simulink model "untitled3"  (R2023a)
settings: Solver=FixedStepAuto  StartTime=0.0  StopTime=3  FixedStep=1e-5  RelTol=1e-3
undefined symbols (not defined in the file): J, KT, La, Ra, UaN
libraries: spsMosfetLib x8, spsDCVoltageSourceLib x2, simulink x2, spsVoltageMeasurementLib x2, spsDCMachineLib x1, sps_lib x1
settings Model: Creator=luand  LastModifiedBy=luand

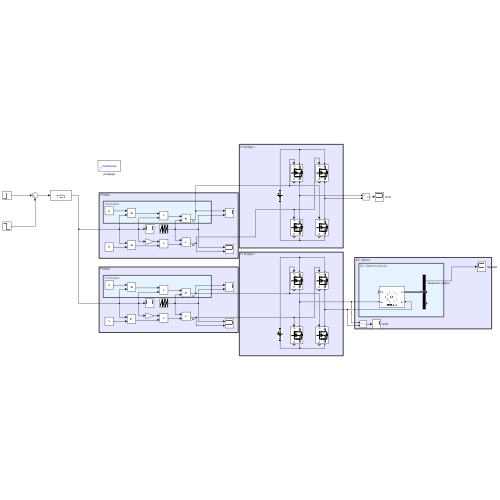
[thumbnail: Simulink's stored preview of the top-level diagram]
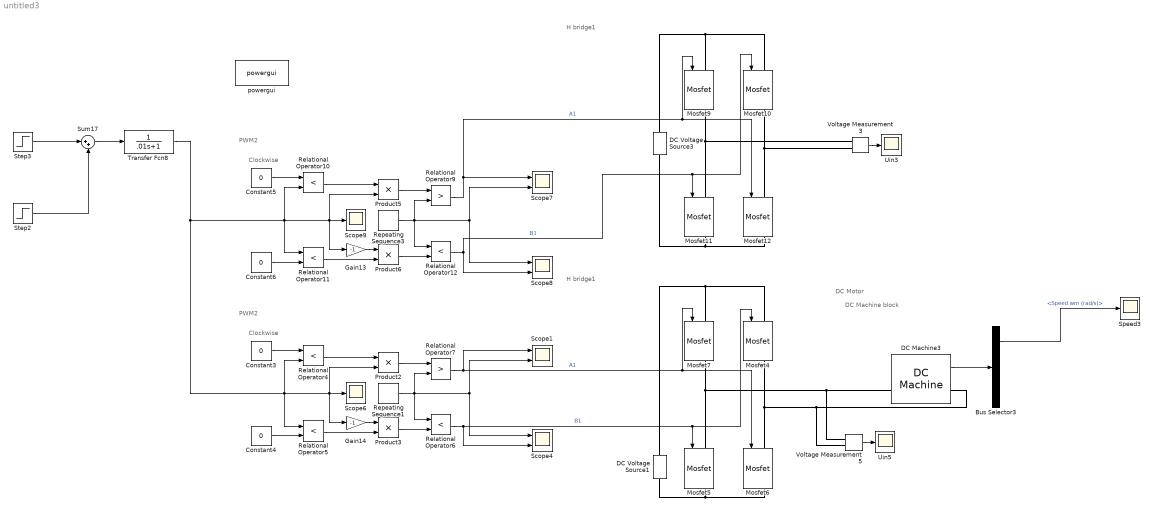
== system untitled3 ==
  note: PWM2
  note: Clockwise
  note: DC Machine block
  note: DC Motor
  note: PWM2
  note: H bridge1
  note: Clockwise
  note: H bridge1
  Bus Selector3 : BusSelector  OutputSignals=Speed wm (rad/s),Armature current ia (A),Electrical torque Te (n m)
  Constant{3..6} (4 alike) : Constant  Value=0
  DC Machine3 : spsDCMachineLib/DC Machine  PresetModel=No  MechanicalLoad=Torque TL  FieldType=Permanent magnet  ShowDetailedParameters=on  MeasurementBus=off  RLa=[ Ra La ]  RLf="[ 240  120]"  Laf=1.8  MachineConstant=Torque constant (N.m/A)  Ke=1.8  Kt=KT  J=J  Bm=0  Tf=0  w0=0  Ifinit=1  TsPowergui=0  TsBlock=-1
  DC Voltage Source1 : spsDCVoltageSourceLib/DC Voltage Source  Amplitude=UaN  Measurements=None
  DC Voltage Source3 : spsDCVoltageSourceLib/DC Voltage Source  Amplitude=UaN  Measurements=None
  Gain13 : Gain  Gain=-1
  Gain14 : Gain  Gain=-1
  Mosfet{4..7,9..12} (8 alike) : spsMosfetLib/Mosfet  Ron=1e-3  Lon=0  Rd=0.01  Vfd=0  IC=0  Rs=1e5  Cs=inf  Measurements=on
  Product{2..3,5..6} (4 alike) : Product
  Relational Operator{4..6,10..12} (6 alike) : RelationalOperator  Operator=<  OutDataTypeStr=boolean  RndMeth=Simplest  InputSameDT=off
  Relational Operator7 : RelationalOperator  Operator=>  OutDataTypeStr=boolean  RndMeth=Simplest  InputSameDT=off
  Relational Operator9 : RelationalOperator  Operator=>  OutDataTypeStr=boolean  RndMeth=Simplest  InputSameDT=off
  Repeating Sequence1 : simulink/Sources/Repeating Sequence  rep_seq_t=[0 1e-3]  rep_seq_y=[0 1]
  Repeating Sequence3 : simulink/Sources/Repeating Sequence  rep_seq_t=[0 1e-3]  rep_seq_y=[0 1]
  Scope{1,4,7..8} (4 alike) : Scope  NumInputPorts=2
  Scope6 : Scope
  Scope9 : Scope
  Speed3 : Scope
  Step2 : Step  After=-1  SampleTime=0
  Step3 : Step  Time=0  After=.5  SampleTime=0
  Sum17 : Sum  Inputs=|++
  Transfer Fcn8 : TransferFcn  Denominator=[.01 1]
  Uin3 : Scope
  Uin5 : Scope
  Voltage Measurement3 : spsVoltageMeasurementLib/Voltage Measurement  PhasorSimulation=off  OutputType=Complex  PSBequivalent=0
  Voltage Measurement5 : spsVoltageMeasurementLib/Voltage Measurement  PhasorSimulation=off  OutputType=Complex  PSBequivalent=0
  powergui : sps_lib/powergui  Priority=1  SimulationMode=Continuous  SampleTime=1e-5  frequency=60  Iterations=50  frequencyindice=0  Pbase=100e6  ErrMax=1e-4  UnitsV=kV  UnitsW=MW  buscounter=0  FunctionMessages=off  echomessages=off  EnableUseOfTLC=off  CurrentSourceSwitches=off  DisableSnubberDevices=off  DisableRonSwitches=off  DisableVfSwitches=off  DisplayEquations=off  AutomaticDiscreteSolvers=off  SolverType=Tustin/Backward Euler (TBE)  Interpol=off  ExternalGateDelay=off  methode=off  Ts=100  x0status=blocks  SPID=on  SwTol=0  HookPort=off  NonlinearTolerance=1e-4  nMaxIteration=100  ContinueOnMaxIteration=off  RestoreLinks=warning  ResistiveCurrentMeasurement=off  Frange=[0:2:500]  Ylog=off  Xlog=on  ShowGrid=off  save=off  variable=ZData  structure=0  ZoomFFT=off  StartTime=0.0  cycles=1  DisplayStyle=1  fundamental=60  FreqAxis=off  MaxFrequency=1000  frequencyindicesteady=1  RmsSteady=1  display=off
  wires:
  Transfer Fcn8/1 -> Relational Operator4/2, Scope6/1, Gain14/1, Product2/2, Relational Operator5/1, Relational Operator11/1, Product5/2, Gain13/1, Scope9/1, Relational Operator10/2
  Step2/1 -> Sum17/2
  DC Machine3/1 -> Bus Selector3/1
  Relational Operator9/1 -> Scope7/1, Mosfet9/1, Mosfet12/1  "A1"
  Sum17/1 -> Transfer Fcn8/1
  Bus Selector3/1 -> Speed3/1  "<Speed wm (rad/s)>"
  Product3/1 -> Relational Operator6/2
  Constant4/1 -> Relational Operator5/2
  Constant6/1 -> Relational Operator11/2
  Voltage Measurement3/1 -> Uin3/1
  Product5/1 -> Relational Operator9/1
  Relational Operator6/1 -> Mosfet5/1, Mosfet4/1, Scope4/2  "B1"
  Relational Operator4/1 -> Product2/1
  Step3/1 -> Sum17/1
  Constant3/1 -> Relational Operator4/1
  Gain14/1 -> Product3/1
  Repeating Sequence3/1 -> Relational Operator9/2, Relational Operator12/1, Scope7/2, Scope8/1
  Constant5/1 -> Relational Operator10/1
  Voltage Measurement5/1 -> Uin5/1
  Relational Operator5/1 -> Product3/2
  Repeating Sequence1/1 -> Relational Operator6/1, Scope4/1, Scope1/2, Relational Operator7/2
  Relational Operator10/1 -> Product5/1
  Gain13/1 -> Product6/1
  Relational Operator7/1 -> Mosfet6/1, Mosfet7/1, Scope1/1  "A1"
  Relational Operator12/1 -> Scope8/2, Mosfet11/1, Mosfet10/1  "B1"
  Relational Operator11/1 -> Product6/2
  Product2/1 -> Relational Operator7/1
  Product6/1 -> Relational Operator12/2
  connections:
  Mosfet7/LConn1 -- Mosfet4/LConn1 -- DC Voltage Source1/RConn1
  Mosfet9/LConn1 -- DC Voltage Source3/RConn1 -- Mosfet10/LConn1
  DC Machine3/LConn1 -- Voltage Measurement5/LConn1 -- Mosfet7/RConn1 -- Mosfet5/LConn1
  Mosfet6/RConn1 -- DC Voltage Source1/LConn1 -- Mosfet5/RConn1
  DC Machine3/RConn1 -- Voltage Measurement5/LConn2 -- Mosfet4/RConn1 -- Mosfet6/LConn1
  Voltage Measurement3/LConn2 -- Mosfet10/RConn1 -- Mosfet12/LConn1
  Mosfet12/RConn1 -- Mosfet11/RConn1 -- DC Voltage Source3/LConn1
  Mosfet11/LConn1 -- Mosfet9/RConn1 -- Voltage Measurement3/LConn1
